simulink model "rlc_serie_passa_faixa"  (R2020a)
settings: Solver=VariableStepAuto  StartTime=0.0  StopTime=0.5  RelTol=1e-3
values from neighbouring files (symbols this model uses):
  C = 0.001    [Variaveis.mat]
  L = 0.1    [Variaveis.mat]
  R = 50    [Variaveis.mat]
libraries: powerlib x7
settings Model: Creator=ed385  LastModifiedBy=Win10

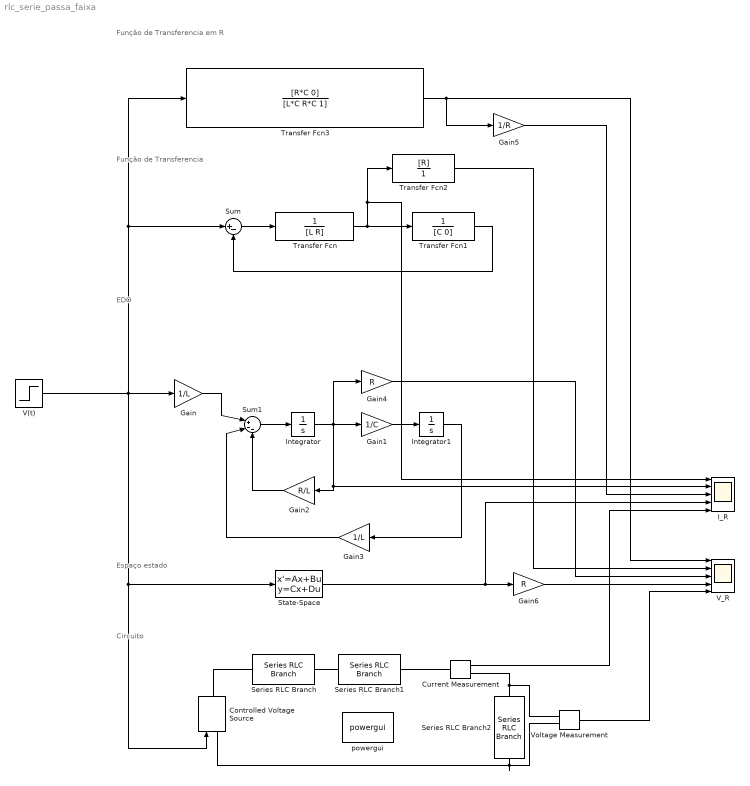
== system rlc_serie_passa_faixa ==
  note: Circuito
  note: Espaço estado
  note: Função de Transferencia
  note: EDO
  note: Função de Transferencia em R
  Controlled Voltage Source : powerlib/Electrical Sources/Controlled Voltage Source  Initialize=on  Source_Type=AC  Amplitude=0  Phase=0  Frequency=0  Measurements=None
  Current Measurement : powerlib/Measurements/Current Measurement  PhasorSimulation=off  OutputType=Complex  PSBequivalent=0
  Gain : Gain  Gain=1/L
  Gain1 : Gain  Gain=1/C
  Gain2 : Gain  Gain=R/L
  Gain3 : Gain  Gain=1/L
  Gain4 : Gain  Gain=R
  Gain5 : Gain  Gain=1/R
  Gain6 : Gain  Gain=R
  I_R : Scope  NumInputPorts=5
  Integrator : Integrator
  Integrator1 : Integrator
  Series RLC Branch : powerlib/Elements/Series RLC Branch  LConnTagsString=__new0  RConnTagsString=__new0  BranchType=L  Resistance=R  Inductance=L  SetiL0=off  InitialCurrent=0  Capacitance=1e-6  Setx0=off  InitialVoltage=0  Measurements=None
  Series RLC Branch1 : powerlib/Elements/Series RLC Branch  LConnTagsString=__new0  RConnTagsString=__new0  BranchType=C  Resistance=R  Inductance=L  SetiL0=off  InitialCurrent=0  Capacitance=C  Setx0=off  InitialVoltage=0  Measurements=None
  Series RLC Branch2 : powerlib/Elements/Series RLC Branch  LConnTagsString=__new0  RConnTagsString=__new0  BranchType=R  Resistance=R  Inductance=L  SetiL0=off  InitialCurrent=0  Capacitance=C  Setx0=off  InitialVoltage=0  Measurements=None
  State-Space : StateSpace  A=[-R/L -1/L;1/C 0]  B=[1/L;0]  C=[1 0;0 1]  D=[0;0]  InitialCondition=0
  Sum : Sum  Inputs=|+-
  Sum1 : Sum  Inputs=|+--
  Transfer Fcn : TransferFcn  Denominator=[L R]
  Transfer Fcn1 : TransferFcn  Denominator=[C 0]
  Transfer Fcn2 : TransferFcn  Numerator=[R]  Denominator=[1]
  Transfer Fcn3 : TransferFcn  Numerator=[R*C 0]  Denominator=[L*C R*C 1]
  V(t) : Step  Time=0  After=10  SampleTime=0
  V_R : Scope  NumInputPorts=5
  Voltage Measurement : powerlib/Measurements/Voltage Measurement  PhasorSimulation=off  OutputType=Complex  PSBequivalent=0
  powergui : powerlib/powergui  Priority=1  SimulationMode=Continuous  SampleTime=50e-6  frequency=60  Iterations=50  frequencyindice=0  Pbase=100e6  ErrMax=1e-4  UnitsV=kV  UnitsW=MW  buscounter=0  FunctionMessages=off  echomessages=off  EnableUseOfTLC=off  CurrentSourceSwitches=off  DisableSnubberDevices=off  DisableRonSwitches=off  DisableVfSwitches=off  DisplayEquations=off  AutomaticDiscreteSolvers=off  SolverType=Tustin/Backward Euler (TBE)  Interpol=off  ExternalGateDelay=off  methode=off  Ts=10  x0status=blocks  SPID=off  SwTol=0  HookPort=off  NonlinearTolerance=1e-4  nMaxIteration=100  ContinueOnMaxIteration=off  RestoreLinks=warning  ResistiveCurrentMeasurement=off  Frange=[0:2:500]  Ylog=off  Xlog=on  ShowGrid=off  save=off  variable=ZData  structure=0  ZoomFFT=off  StartTime=0.0  cycles=1  DisplayStyle=1  fundamental=60  FreqAxis=off  MaxFrequency=1000  frequencyindicesteady=1  RmsSteady=1  display=off
  wires:
  V(t)/1 -> Transfer Fcn3/1, Sum/1, State-Space/1, Controlled Voltage Source/1, Gain/1
  Sum/1 -> Transfer Fcn/1
  Transfer Fcn/1 -> Transfer Fcn2/1, I_R/1, Transfer Fcn1/1
  Transfer Fcn1/1 -> Sum/2
  State-Space/1 -> Gain6/1, I_R/4
  Gain/1 -> Sum1/1
  Sum1/1 -> Integrator/1
  Gain1/1 -> Integrator1/1
  Integrator/1 -> I_R/2, Gain2/1, Gain4/1, Gain1/1
  Gain2/1 -> Sum1/3
  Gain3/1 -> Sum1/2
  Integrator1/1 -> Gain3/1
  Gain4/1 -> V_R/3
  Transfer Fcn2/1 -> V_R/2
  Transfer Fcn3/1 -> V_R/1, Gain5/1
  Gain5/1 -> I_R/3
  Gain6/1 -> V_R/4
  Current Measurement/1 -> I_R/5
  Voltage Measurement/1 -> V_R/5
  connections:
  Voltage Measurement/LConn2 -- Series RLC Branch2/RConn1 -- Controlled Voltage Source/LConn1
  Series RLC Branch2/LConn1 -- Current Measurement/RConn1 -- Voltage Measurement/LConn1
  Current Measurement/LConn1 -- Series RLC Branch1/RConn1
  Series RLC Branch1/LConn1 -- Series RLC Branch/RConn1
  Series RLC Branch/LConn1 -- Controlled Voltage Source/RConn1
